simulink subsystem "fullCycleDocked_cl"  (R2022a)
settings: Solver=VariableStepAuto  StartTime=0.0  StopTime=10.0  RelTol=1e-3
settings Model: Creator=sam3b  LastModifiedBy=lhill8
settings SolverCC: AlgebraicLoopSolver=TrustRegion
settings DebuggingCC: UnconnectedInputMsg=warning  UnconnectedOutputMsg=warning  UnconnectedLineMsg=warning  SFMachineParentedDataDiag=warning

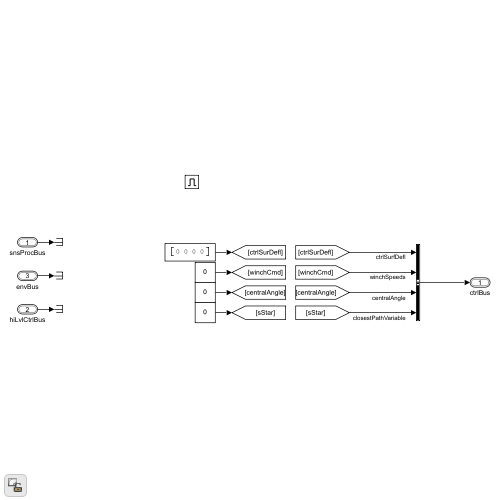
[thumbnail: Simulink's stored preview of the top-level diagram]
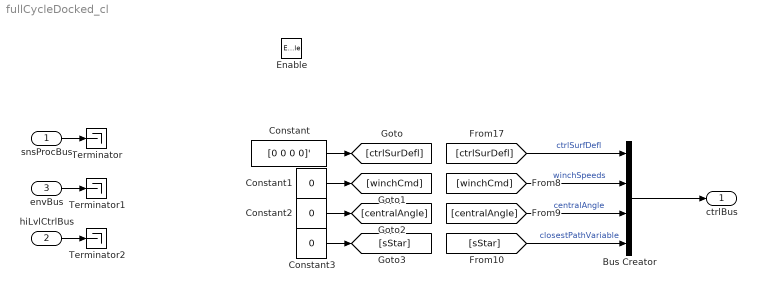
== system fullCycleDocked_cl ==
  snsProcBus : Inport  OutDataTypeStr=Bus: sensorsProcessingBus
  hiLvlCtrlBus : Inport  Port=2  OutDataTypeStr=Bus: hiLvlCtrlBus
  envBus : Inport  Port=3  OutDataTypeStr=Bus: envBus
  Enable : EnablePort
  Bus Creator : BusCreator  Inputs=4  OutDataTypeStr=Bus: fltCtrlBus
      settings: InheritFromInputs=off
  Constant : Constant  Value=[0 0 0 0]'
  Constant1 : Constant  Value=0
  Constant2 : Constant  Value=0
  Constant3 : Constant  Value=0
  Terminator : Terminator
  Terminator1 : Terminator
  Terminator2 : Terminator
  ctrlBus : Outport  OutDataTypeStr=Bus: fltCtrlBus  VectorParamsAs1DForOutWhenUnconnected=off
  wires:
  envBus/1 -> Terminator1/1
  Constant2/1 -> [centralAngle]
  [ctrlSurDefl] -> Bus Creator/1  "ctrlSurfDefl"
  Constant3/1 -> [sStar]
  Constant1/1 -> [winchCmd]
  hiLvlCtrlBus/1 -> Terminator2/1
  Constant/1 -> [ctrlSurDefl]
  [sStar] -> Bus Creator/4  "closestPathVariable"
  snsProcBus/1 -> Terminator/1
  [centralAngle] -> Bus Creator/3  "centralAngle"
  [winchCmd] -> Bus Creator/2  "winchSpeeds"
  Bus Creator/1 -> ctrlBus/1
